simulink model "BattU_DD"  (R2016b)
settings: configuration reference "CodeGenConfigSet" (kept outside this file)
values from neighbouring files (symbols this model uses):
  BattU_tiMaxDefDeb_C = Calibration.Parameter    [init_BattU_DD.m]
  BattU_tiMaxOKDeb_C = Calibration.Parameter    [init_BattU_DD.m]
  BattU_tiMinDefDeb_C = Calibration.Parameter    [init_BattU_DD.m]
  BattU_tiMinOKDeb_C = Calibration.Parameter    [init_BattU_DD.m]
  BattU_tiPhysRngHiDefDeb_C = Calibration.Parameter    [init_BattU_DD.m]
  BattU_tiPhysRngHiOKDeb_C = Calibration.Parameter    [init_BattU_DD.m]
  BattU_tiPhysRngLoDefDeb_C = Calibration.Parameter    [init_BattU_DD.m]
  BattU_tiPhysRngLoOKDeb_C = Calibration.Parameter    [init_BattU_DD.m]
  BattU_uPhysRngMax_C = Calibration.Parameter    [init_BattU_DD.m]
  BattU_uPhysRngMin_C = Calibration.Parameter    [init_BattU_DD.m]
  BattU_uSRCMax_C = Calibration.Parameter    [init_BattU_DD.m]
  BattU_uSRCMin_C = Calibration.Parameter    [init_BattU_DD.m]
  BattU_uTransf_CUR = Calibration.Parameter    [init_BattU_DD.m]
  BattU_uTransf_CURX = Calibration.Parameter    [init_BattU_DD.m]
undefined symbols (not defined in the file or in its folder): BattU_DD_DT
libraries: CXLib x12
settings Model: Creator=Administrator  LastModifiedBy=wangrui
settings ConfigSetRef: SourceLocation=Base Workspace

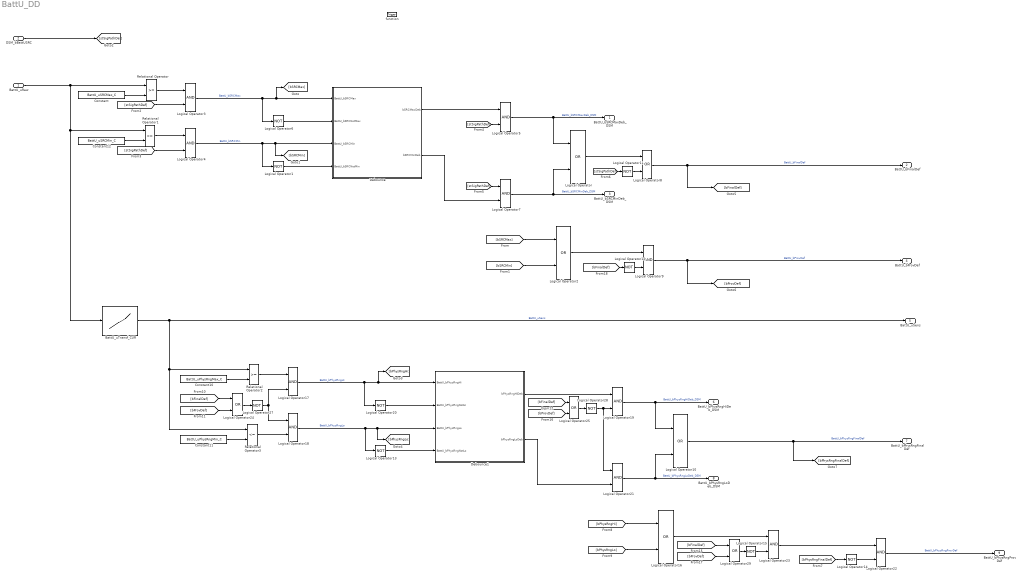
== system BattU_DD ==
  BattU_uRaw : Inport  Tag=mv  Description=Battery voltage before defect detection and handling  OutMin=0  OutMax=5000  OutDataTypeStr=Ad_mv
  DSM_bBattUSRC : Inport  Description=Status of FId_BattUSRC  Port=2  OutMin=0  OutMax=1  OutDataTypeStr=boolean
  function : TriggerPort  TriggerType=function-call  VariantControl=Variant
  BattU_uTransf_CUR : Lookup_n-D  NumberOfTableDimensions=1  BreakpointsForDimension1=BattU_uTransf_CURX  IndexSearchMethod=Linear search  BeginIndexSearchUsingPreviousIndexResult=on  UseOneInputPortForAllInputData=on  Table=BattU_uTransf_CUR  ExtrapMethod=Clip  UseLastTableValue=on  InternalRulePriority=Speed  OutDataTypeStr=Inherit: Inherit via back propagation  SaturateOnIntegerOverflow=on
  Constant : Constant  Value=BattU_uSRCMax_C
  Constant10 : Constant  Value=BattU_uPhysRngMax_C
  Constant11 : Constant  Value=BattU_uPhysRngMin_C
  Constant12 : Constant  Value=BattU_uSRCMin_C
  Debounce : Subsystem
  Debounce1 : Subsystem
  Logical Operator{,2,8,10,16} (5 alike) : Logic  Operator=OR  AllPortsSameDT=off  OutDataTypeStr=boolean
  Logical Operator{1,6,11..15,20,27..28} (10 alike) : Logic  Operator=NOT  AllPortsSameDT=off  OutDataTypeStr=boolean
  Logical Operator{3..5,7,9,17..19,21..23} (11 alike) : Logic  AllPortsSameDT=off  OutDataTypeStr=boolean
  Logical Operator24 : Logic  Operator=OR  OutDataTypeStr=boolean
  Logical Operator25 : Logic  Operator=OR  OutDataTypeStr=boolean
  Logical Operator29 : Logic  Operator=OR  OutDataTypeStr=boolean
  Relational Operator : RelationalOperator  OutDataTypeStr=boolean  RndMeth=Nearest  InputSameDT=on
  Relational Operator1 : RelationalOperator  Operator=<=  OutDataTypeStr=boolean  RndMeth=Nearest  InputSameDT=on
  Relational Operator2 : RelationalOperator  OutDataTypeStr=boolean  RndMeth=Nearest  InputSameDT=on
  Relational Operator3 : RelationalOperator  Operator=<=  OutDataTypeStr=boolean  RndMeth=Nearest  InputSameDT=on
  BattU_bSRCMaxDeb_DSM : Outport  Description=status of BattU_bSRCMaxDeb  OutMin=0  OutMax=1  OutDataTypeStr=boolean
  BattU_bFinalDef : Outport  Description=Status Sensor of the battery voltage finally defect  Port=2  OutMin=0  OutMax=1  OutDataTypeStr=boolean
  BattU_bSRCMinDeb_DSM : Outport  Description=status of BattU_bSRCMinDeb  Port=3  OutMin=0  OutMax=1  OutDataTypeStr=boolean
  BattU_bProvDef : Outport  Description=Status Sensor of the battery voltage temporary defect  Port=4  OutMin=0  OutMax=1  OutDataTypeStr=boolean
  BattU_uSens : Outport  Tag=mv  Description=Sensed battery voltage  Port=5  OutMin=0  OutMax=50000  OutDataTypeStr=Battery_mv
  BattU_bPhysRngHiDeb_DSM : Outport  Description=status of BattU_bPhysRngHiDeb  Port=6  OutMin=0  OutMax=1  OutDataTypeStr=boolean
  BattU_bPhysRngFinalDef : Outport  Description="Status Sensor of the  battery voltage physical Signal range check finally defect"  Port=7  OutMin=0  OutMax=1  OutDataTypeStr=boolean
  BattU_bPhysRngLoDeb_DSM : Outport  Description=status of BattU_bPhysRngLoDeb  Port=8  OutMin=0  OutMax=1  OutDataTypeStr=boolean
  BattU_bPhysRngProvDef : Outport  Description=Status Sensor of the battery voltage physical Signal range check temporary defect  Port=9  OutMin=0  OutMax=1  OutDataTypeStr=boolean
  wires:
  Constant/1 -> Relational Operator/2
  Logical Operator3/1 -> Logical Operator6/1, [bSRCMax], Debounce/1(BattU_bSRCMax)  "BattU_bSRCMax"
  Constant12/1 -> Relational Operator1/2
  Logical Operator4/1 -> Logical Operator1/1, [bSRCMin], Debounce/3(BattU_bSRCMin)  "BattU_bSRCMin"
  Logical Operator5/1 -> BattU_bSRCMaxDeb_DSM/1, Logical Operator/1  "BattU_bSRCMaxDeb_DSM"
  Logical Operator7/1 -> BattU_bSRCMinDeb_DSM/1, Logical Operator/2  "BattU_bSRCMinDeb_DSM"
  [bSRCMax] -> Logical Operator2/1
  [bSRCMin] -> Logical Operator2/2
  DSM_bBattUSRC/1 -> [stSigPathDef]
  Relational Operator/1 -> Logical Operator3/1
  [stSigPathDef] -> Logical Operator3/2
  Relational Operator1/1 -> Logical Operator4/1
  [stSigPathDef] -> Logical Operator4/2
  [stSigPathDef] -> Logical Operator5/2
  [stSigPathDef] -> Logical Operator7/1
  Logical Operator/1 -> Logical Operator8/1
  [stSigPathDef] -> Logical Operator11/1
  Logical Operator2/1 -> Logical Operator9/1
  [bFinalDef] -> Logical Operator12/1
  Logical Operator8/1 -> BattU_bFinalDef/1, [bFinalDef]  "BattU_bFinalDef"
  Logical Operator9/1 -> BattU_bProvDef/1, [bProvDef]  "BattU_bProvDef"
  Logical Operator11/1 -> Logical Operator8/2
  Logical Operator12/1 -> Logical Operator9/2
  BattU_uRaw/1 -> BattU_uTransf_CUR/1, Relational Operator1/1, Relational Operator/1
  Logical Operator6/1 -> Debounce/2(BattU_bSRCNotMax)
  Logical Operator1/1 -> Debounce/4(BattU_bSRCNotMin)
  Debounce/1(bSRCMaxDeb) -> Logical Operator5/1
  Debounce/2(bSRCMinDeb) -> Logical Operator7/2
  BattU_uTransf_CUR/1 -> BattU_uSens/1, Relational Operator3/1, Relational Operator2/1  "BattU_uSens"
  Constant10/1 -> Relational Operator2/2
  Logical Operator17/1 -> Logical Operator20/1, [bPhysRngHi], Debounce1/1(BattU_bPhysRngHi)  "BattU_bPhysRngHi"
  Constant11/1 -> Relational Operator3/2
  Logical Operator18/1 -> Logical Operator13/1, [bPhysRngLo], Debounce1/3(BattU_bPhysRngLo)  "BattU_bPhysRngLo"
  Logical Operator19/1 -> BattU_bPhysRngHiDeb_DSM/1, Logical Operator10/1  "BattU_bPhysRngHiDeb_DSM"
  Logical Operator21/1 -> BattU_bPhysRngLoDeb_DSM/1, Logical Operator10/2  "BattU_bPhysRngLoDeb_DSM"
  [bPhysRngHi] -> Logical Operator16/1
  [bPhysRngLo] -> Logical Operator16/2
  Relational Operator2/1 -> Logical Operator17/1
  Logical Operator24/1 -> Logical Operator27/1
  Logical Operator25/1 -> Logical Operator28/1
  Logical Operator16/1 -> Logical Operator23/1
  Logical Operator10/1 -> BattU_bPhysRngFinalDef/1, [bPhysRngFinalDef]  "BattU_bPhysRngFinalDef"
  Logical Operator15/1 -> Logical Operator23/2
  Logical Operator20/1 -> Debounce1/2(BattU_bPhysRngNotHi)
  Logical Operator13/1 -> Debounce1/4(BattU_bPhysRngNotLo)
  Debounce1/1(bPhysRngHiDeb) -> Logical Operator19/1
  Relational Operator3/1 -> Logical Operator18/2
  [bFinalDef] -> Logical Operator24/1
  [bProvDef] -> Logical Operator24/2
  [bFinalDef] -> Logical Operator25/1
  [bProvDef] -> Logical Operator25/2
  Debounce1/2(bPhysRngLoDeb) -> Logical Operator21/2
  Logical Operator27/1 -> Logical Operator18/1, Logical Operator17/2
  Logical Operator28/1 -> Logical Operator21/1, Logical Operator19/2
  [bFinalDef] -> Logical Operator29/1
  [bProvDef] -> Logical Operator29/2
  Logical Operator29/1 -> Logical Operator15/1
  [bPhysRngFinalDef] -> Logical Operator14/1
  Logical Operator14/1 -> Logical Operator22/2
  Logical Operator23/1 -> Logical Operator22/1
  Logical Operator22/1 -> BattU_bPhysRngProvDef/1  "BattU_bPhysRngProvDef"

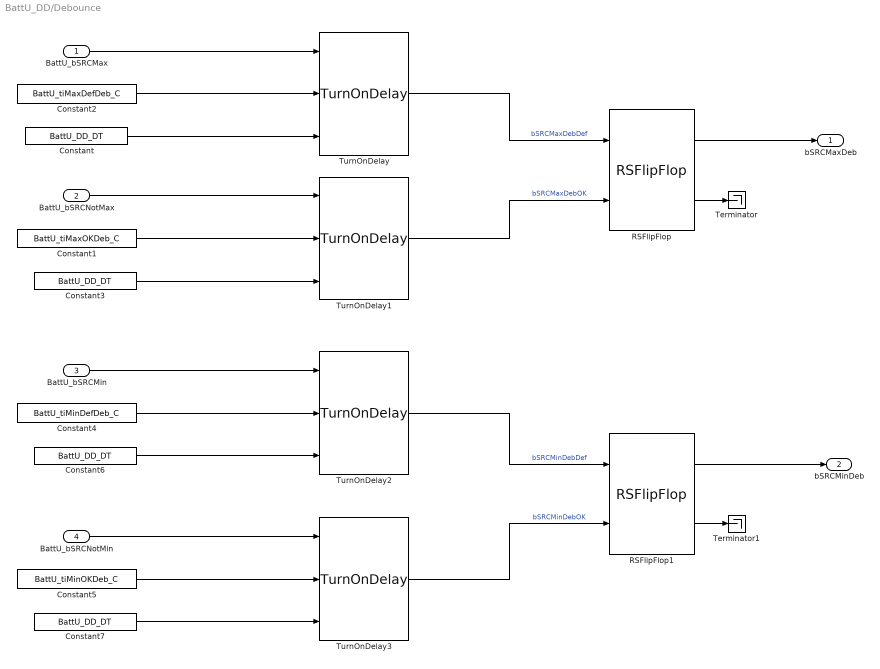
== system BattU_DD/Debounce ==
  BattU_bSRCMax : Inport
  BattU_bSRCNotMax : Inport  Port=2
  BattU_bSRCMin : Inport  Port=3
  BattU_bSRCNotMin : Inport  Port=4
  Constant{,3,6..7} (4 alike) : Constant  Value=BattU_DD_DT  OutDataTypeStr=Inherit: Inherit via back propagation
  Constant1 : Constant  Value=BattU_tiMaxOKDeb_C
  Constant2 : Constant  Value=BattU_tiMaxDefDeb_C
  Constant4 : Constant  Value=BattU_tiMinDefDeb_C
  Constant5 : Constant  Value=BattU_tiMinOKDeb_C
  RSFlipFlop : CXLib/RSFlipFlop
  RSFlipFlop1 : CXLib/RSFlipFlop
  Terminator : Terminator
  Terminator1 : Terminator
  TurnOnDelay{,1..3} (4 alike) : CXLib/TurnOnDelay
  bSRCMaxDeb : Outport
  bSRCMinDeb : Outport  Port=2
  wires:
  RSFlipFlop1/1 -> bSRCMinDeb/1
  RSFlipFlop/1 -> bSRCMaxDeb/1
  TurnOnDelay1/1 -> RSFlipFlop/2  "bSRCMaxDebOK"
  Constant4/1 -> TurnOnDelay2/2
  Constant1/1 -> TurnOnDelay1/2
  Constant2/1 -> TurnOnDelay/2
  TurnOnDelay/1 -> RSFlipFlop/1  "bSRCMaxDebDef"
  BattU_bSRCNotMax/1 -> TurnOnDelay1/1
  BattU_bSRCMin/1 -> TurnOnDelay2/1
  TurnOnDelay2/1 -> RSFlipFlop1/1  "bSRCMinDebDef"
  BattU_bSRCNotMin/1 -> TurnOnDelay3/1
  TurnOnDelay3/1 -> RSFlipFlop1/2  "bSRCMinDebOK"
  Constant5/1 -> TurnOnDelay3/2
  RSFlipFlop/2 -> Terminator/1
  RSFlipFlop1/2 -> Terminator1/1
  BattU_bSRCMax/1 -> TurnOnDelay/1
  Constant/1 -> TurnOnDelay/3
  Constant3/1 -> TurnOnDelay1/3
  Constant6/1 -> TurnOnDelay2/3
  Constant7/1 -> TurnOnDelay3/3

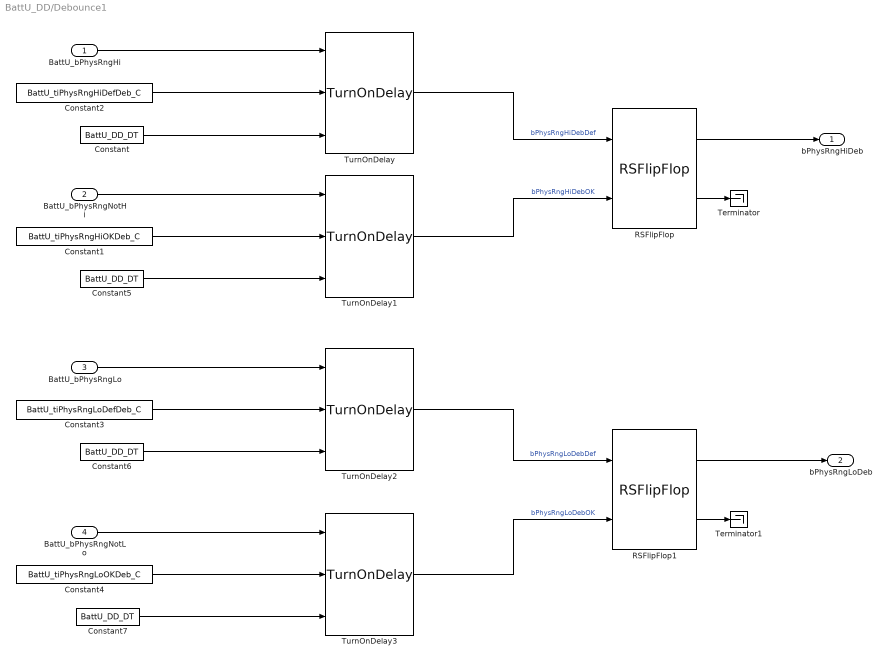
== system BattU_DD/Debounce1 ==
  BattU_bPhysRngHi : Inport
  BattU_bPhysRngNotHi : Inport  Port=2
  BattU_bPhysRngLo : Inport  Port=3
  BattU_bPhysRngNotLo : Inport  Port=4
  Constant{,5..7} (4 alike) : Constant  Value=BattU_DD_DT  OutDataTypeStr=Inherit: Inherit via back propagation
  Constant1 : Constant  Value=BattU_tiPhysRngHiOKDeb_C
  Constant2 : Constant  Value=BattU_tiPhysRngHiDefDeb_C
  Constant3 : Constant  Value=BattU_tiPhysRngLoDefDeb_C
  Constant4 : Constant  Value=BattU_tiPhysRngLoOKDeb_C
  RSFlipFlop : CXLib/RSFlipFlop
  RSFlipFlop1 : CXLib/RSFlipFlop
  Terminator : Terminator
  Terminator1 : Terminator
  TurnOnDelay{,1..3} (4 alike) : CXLib/TurnOnDelay
  bPhysRngHiDeb : Outport
  bPhysRngLoDeb : Outport  Port=2
  wires:
  BattU_bPhysRngHi/1 -> TurnOnDelay/1
  RSFlipFlop1/2 -> Terminator1/1
  RSFlipFlop/2 -> Terminator/1
  Constant4/1 -> TurnOnDelay3/2
  TurnOnDelay3/1 -> RSFlipFlop1/2  "bPhysRngLoDebOK"
  BattU_bPhysRngNotLo/1 -> TurnOnDelay3/1
  TurnOnDelay2/1 -> RSFlipFlop1/1  "bPhysRngLoDebDef"
  BattU_bPhysRngLo/1 -> TurnOnDelay2/1
  BattU_bPhysRngNotHi/1 -> TurnOnDelay1/1
  TurnOnDelay/1 -> RSFlipFlop/1  "bPhysRngHiDebDef"
  Constant2/1 -> TurnOnDelay/2
  Constant1/1 -> TurnOnDelay1/2
  Constant3/1 -> TurnOnDelay2/2
  TurnOnDelay1/1 -> RSFlipFlop/2  "bPhysRngHiDebOK"
  RSFlipFlop/1 -> bPhysRngHiDeb/1
  RSFlipFlop1/1 -> bPhysRngLoDeb/1
  Constant/1 -> TurnOnDelay/3
  Constant5/1 -> TurnOnDelay1/3
  Constant6/1 -> TurnOnDelay2/3
  Constant7/1 -> TurnOnDelay3/3
